simulink model "mdaqdemo_adc"  (R2013a)
settings: Solver=FixedStepDiscrete  StartTime=0.0  StopTime=10.0  RelTol=1e-3
libraries: simulink x1
settings Model: Creator=peselnikmg  LastModifiedBy=skibool
settings DataIOCC: SignalLoggingSaveFormat=ModelDataLogs  SaveOutput=off  SignalLogging=off  DSMLogging=off  SaveTime=off
settings OptimizationCC: InlineParams=on  EnhancedBackFolding=on  OptimizeModelRefInitCode=on  LifeSpan=1
settings HardwareCC: ProdBitPerLong=40  ProdLargestAtomicInteger=Integer  ProdIntDivRoundTo=Zero  ProdEndianess=LittleEndian  ProdHWDeviceType=Texas Instruments->C6000
settings RTWCC: SystemTargetFile=microdaq.tlc  TemplateMakefile=microdaq.tmf  PostCodeGenCommand=microdaq_postcodegen(buildInfo)  Description=MicroDAQ Real-Time Measurement System  GenerateReport=on  ProcessScript=microdaq_make_rtw_hook  IncludeHyperlinkInReport=on  LaunchReport=on
settings CodeAppCC: IgnoreCustomStorageClasses=off
settings STFCustomTargetCC: CodeReplacementLibrary=TI C674x  IncludeMdlTerminateFcn=off  CombineOutputUpdateFcns=on  SuppressErrorStatus=on  ERTCustomFileBanners=on  SupportAbsoluteTime=off  SupportNonFinite=off  SupportComplex=off  SupportContinuousTime=off  SupportNonInlinedSFcns=off  MATLABClassNameForMDSCustomization=Simulink.SoftwareTarget.ERTCustomization  SystemTargetFile=microdaq.tlc
settings ERTTargetCC: CodeReplacementLibrary=TI C674x  GenerateSampleERTMain=off  ParMdlRefBuildCompliant=off  CompOptLevelCompliant=off  ConcurrentExecutionCompliant=off  IncludeMdlTerminateFcn=off  SuppressErrorStatus=on  ERTFirstTimeCompliant=off  SupportAbsoluteTime=off  SupportNonFinite=off  SupportComplex=off  ModelStepFunctionPrototypeControlCompliant=off  CPPClassGenCompliant=off  ERTCustomFileTemplate=microdaq_main.tlc

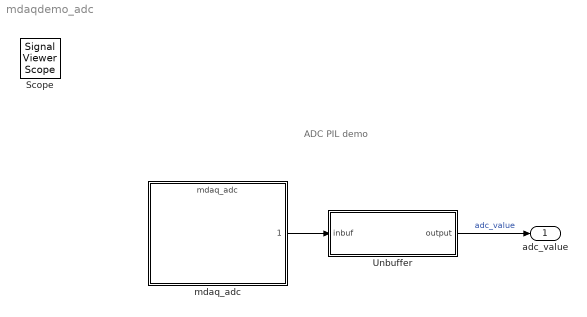
== system mdaqdemo_adc ==
  note: ADC PIL demo
  Unbuffer : Subsystem  TreatAsAtomicUnit=on  mask{BufSize=100, Ts=0.001}
      mask prompts: BufSize "Buffer Size:"; Ts "Sample Time:"
      mask Display:
      | fprintf('Buffer Size: %d\n\n', BufSize);
      | fprintf('\n\nSample Time: %g\n', Ts);
  mdaq_adc : ModelReference  ModelNameDialog=mdaq_adc  SimulationMode=Processor-in-the-loop (PIL)  ModelReferenceVersion=1.61  CopyOfModelName=mdaq_adc  DefaultDataLogging=on
  adc_value : Outport
  Scope : SignalViewerScope  IOType=viewer  NumInputPorts=2  RefreshTime=0.035000
      settings: YMin=-5~-5  YMax=5~5
  wires:
  mdaq_adc/1 -> Unbuffer/1(inbuf)
  Unbuffer/1(output) -> adc_value/1  "adc_value"

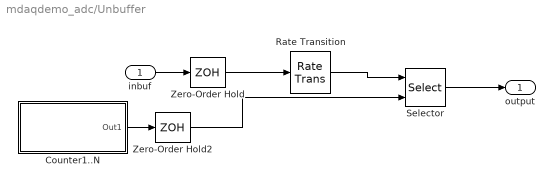
== system mdaqdemo_adc/Unbuffer ==
  inbuf : Inport  SampleTime=Ts
  Counter1..N : Subsystem
      mask Display: disp('Counter')
  Rate Transition : RateTransition
  Selector : Selector  InputPortWidth=BufSize  IndexOptions=Index vector (port)  Indices=[1 3]  OutputSizes=1
  Zero-Order Hold : ZeroOrderHold  SampleTime=BufSize*Ts
  Zero-Order Hold2 : ZeroOrderHold  SampleTime=Ts
  output : Outport
  wires:
  Counter1..N/1(Out1) -> Zero-Order Hold2/1
  Zero-Order Hold2/1 -> Selector/2
  inbuf/1 -> Zero-Order Hold/1
  Selector/1 -> output/1
  Zero-Order Hold/1 -> Rate Transition/1
  Rate Transition/1 -> Selector/1

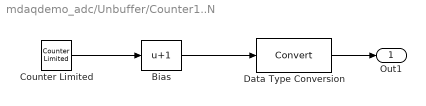
== system mdaqdemo_adc/Unbuffer/Counter1..N ==
  Bias : Bias  Bias=1
  Counter Limited : simulink/Sources/Counter Limited  uplimit=BufSize-1  tsamp=-1
  Data Type Conversion : DataTypeConversion
  Out1 : Outport
  wires:
  Data Type Conversion/1 -> Out1/1
  Bias/1 -> Data Type Conversion/1
  Counter Limited/1 -> Bias/1
